simulink model "model"  (R2023a)
settings: Solver=VariableStepAuto  StartTime=0.0  StopTime=300  RelTol=1e-3
values from neighbouring files (symbols this model uses):
  r0 = unitToMJframe(r0)    [setup.m]
  r1 = unitToMJframe(r1)    [setup.m]
  r2 = unitToMJframe(r2)    [setup.m]
  r3 = unitToMJframe(r3)    [setup.m]
libraries: mjLib x4, sharedutil x4, sharedtransform x4
settings Model: PacingRate=4  Creator=manoj  LastModifiedBy=manoj

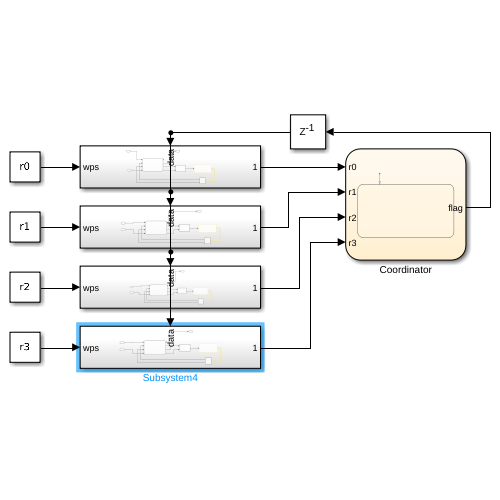
[thumbnail: Simulink's stored preview of the top-level diagram]
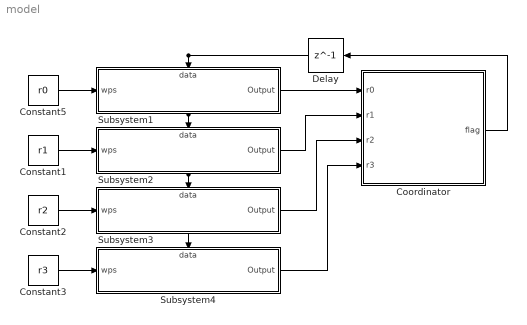
== system model ==
  Constant1 : Constant  Value=r1
  Constant2 : Constant  Value=r2
  Constant3 : Constant  Value=r3
  Constant5 : Constant  Value=r0
  Coordinator : Stateflow chart  TreatAsAtomicUnit=on
  Delay : Delay  DelayLength=1
  Subsystem1 : Subsystem
      settings: PortSchema="{\"entries\":[{\"content\":{\"sides\":[{\"content\":{\"connectorIds\":[\"In1\"]},\"type\":\"ConnectorPlacement.EquallySpacedRectSide\",\"uuid\":\"b8d0416c-6ae9-40e7-8587-4b4901c80a66\"},{\"content\":{\"connectorIds\":[\"Out1\"],\"side\":\"RIGHT\"},\"type\":\"ConnectorPlacement.EquallySpacedRectSide\",\"uuid\":\"eb8da2dc-17d6-409c-8414-2a6f0851cca1\"},{\"content\":{\"connectorIds\":[\"In2\"],\"side\":\"TOP\"},\"type\":\"ConnectorPlacement.EquallySpacedRectSide\",\"uuid\":\"007649e1-b7d1-46e6-9a26-22c717d3ea9f\"}]},\"type\":\"ConnectorPlacement.EquallySpacedConnector\",\"uuid\":\"2131bbaa-72b6-47e6-bef9-d625e80c0564\"}],\"packageUris\":[\"http://schema.mathworks.com/mf0/Connector/R2020b\"],\"version\":\"1.0\"}"
  Subsystem2 : Subsystem
      settings: PortSchema="{\"entries\":[{\"content\":{\"sides\":[{\"content\":{\"connectorIds\":[\"In1\"]},\"type\":\"ConnectorPlacement.EquallySpacedRectSide\",\"uuid\":\"b8d0416c-6ae9-40e7-8587-4b4901c80a66\"},{\"content\":{\"connectorIds\":[\"Out1\"],\"side\":\"RIGHT\"},\"type\":\"ConnectorPlacement.EquallySpacedRectSide\",\"uuid\":\"eb8da2dc-17d6-409c-8414-2a6f0851cca1\"},{\"content\":{\"connectorIds\":[\"In2\"],\"side\":\"TOP\"},\"type\":\"ConnectorPlacement.EquallySpacedRectSide\",\"uuid\":\"007649e1-b7d1-46e6-9a26-22c717d3ea9f\"}]},\"type\":\"ConnectorPlacement.EquallySpacedConnector\",\"uuid\":\"2131bbaa-72b6-47e6-bef9-d625e80c0564\"}],\"packageUris\":[\"http://schema.mathworks.com/mf0/Connector/R2020b\"],\"version\":\"1.0\"}"
  Subsystem3 : Subsystem
      settings: PortSchema="{\"entries\":[{\"content\":{\"sides\":[{\"content\":{\"connectorIds\":[\"In1\"]},\"type\":\"ConnectorPlacement.EquallySpacedRectSide\",\"uuid\":\"b8d0416c-6ae9-40e7-8587-4b4901c80a66\"},{\"content\":{\"connectorIds\":[\"Out1\"],\"side\":\"RIGHT\"},\"type\":\"ConnectorPlacement.EquallySpacedRectSide\",\"uuid\":\"eb8da2dc-17d6-409c-8414-2a6f0851cca1\"},{\"content\":{\"connectorIds\":[\"In2\"],\"side\":\"TOP\"},\"type\":\"ConnectorPlacement.EquallySpacedRectSide\",\"uuid\":\"007649e1-b7d1-46e6-9a26-22c717d3ea9f\"}]},\"type\":\"ConnectorPlacement.EquallySpacedConnector\",\"uuid\":\"2131bbaa-72b6-47e6-bef9-d625e80c0564\"}],\"packageUris\":[\"http://schema.mathworks.com/mf0/Connector/R2020b\"],\"version\":\"1.0\"}"
  Subsystem4 : Subsystem
      settings: PortSchema="{\"entries\":[{\"content\":{\"sides\":[{\"content\":{\"connectorIds\":[\"In1\"]},\"type\":\"ConnectorPlacement.EquallySpacedRectSide\",\"uuid\":\"b8d0416c-6ae9-40e7-8587-4b4901c80a66\"},{\"content\":{\"connectorIds\":[\"Out1\"],\"side\":\"RIGHT\"},\"type\":\"ConnectorPlacement.EquallySpacedRectSide\",\"uuid\":\"eb8da2dc-17d6-409c-8414-2a6f0851cca1\"},{\"content\":{\"connectorIds\":[\"In2\"],\"side\":\"TOP\"},\"type\":\"ConnectorPlacement.EquallySpacedRectSide\",\"uuid\":\"007649e1-b7d1-46e6-9a26-22c717d3ea9f\"}]},\"type\":\"ConnectorPlacement.EquallySpacedConnector\",\"uuid\":\"2131bbaa-72b6-47e6-bef9-d625e80c0564\"}],\"packageUris\":[\"http://schema.mathworks.com/mf0/Connector/R2020b\"],\"version\":\"1.0\"}"
  wires:
  Constant5/1 -> Subsystem1/1(wps)
  Constant1/1 -> Subsystem2/1(wps)
  Constant2/1 -> Subsystem3/1(wps)
  Constant3/1 -> Subsystem4/1(wps)
  Coordinator/1(flag) -> Delay/1
  Subsystem1/1(Output) -> Coordinator/1(r0)
  Subsystem2/1(Output) -> Coordinator/2(r1)
  Subsystem3/1(Output) -> Coordinator/3(r2)
  Subsystem4/1(Output) -> Coordinator/4(r3)
  Delay/1 -> Subsystem1/2(data), Subsystem4/2(data), Subsystem3/2(data), Subsystem2/2(data)

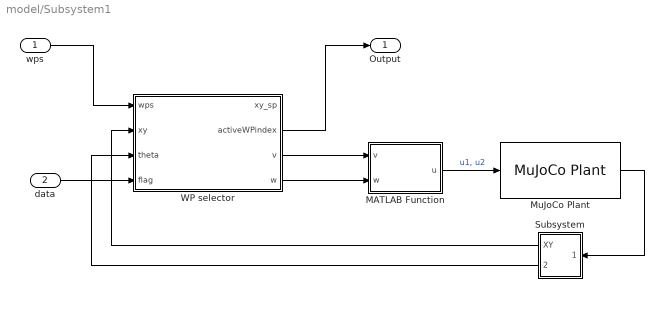
== system model/Subsystem1 ==
  wps : Inport
  data : Inport  Port=2
  MATLAB Function : MATLAB Function  TreatAsAtomicUnit=on
  MuJoCo Plant : mjLib/MuJoCo Plant  controlBus=[]  sensorBus=mj_bus_sensor_7979902499018342666  controlLength=[]  sensorLength=[]  rgbLength=[]  depthLength=[]  sampleTime=0.003  xmlFileRel=/home/manoj/work/courses/Multi_robot_centralized_planning/mujoco/mjxml/testClawbot.xml  xmlFile=/home/manoj/work/courses/Multi_robot_centralized_planning/mujoco/mjxml/testClawbot.xml  renderingType=Global  vsync=off  visualFPS=60  zoomLevel=1  znear=0.067117  zfar=335.5848  cameraSampleTime=0.020  rgbOutOption=on  depthOutOption=on  controlInterfaceType=Vector
      settings: SourceProductName=MuJoCo Simulator
  Subsystem : Subsystem
  WP selector : Stateflow chart  TreatAsAtomicUnit=on
      settings: PortSchema="{\"entries\":[{\"content\":{\"sides\":[{\"content\":{\"connectorIds\":[\"In1\",\"In2\",\"In3\",\"In4\"]},\"type\":\"ConnectorPlacement.EquallySpacedRectSide\",\"uuid\":\"c1ca6372-0066-48a0-9bc3-46210ce06805\"},{\"content\":{\"connectorIds\":[\"Out1\",\"Out2\",\"Out4\",\"Out3\"],\"side\":\"RIGHT\"},\"type\":\"ConnectorPlacement.EquallySpacedRectSide\",\"uuid\":\"5093fe73-baf8-4ce0-b37a-f548b4260345\"},{\"content\":{\"side\":\"TOP\"},\"type\":\"ConnectorPlacement.EquallySpacedRectSide\",\"uuid\":\"dd012d01-db43-40b1-a5e6-c3bf94706175\"}]},\"type\":\"ConnectorPlacement.EquallySpacedConnector\",\"uuid\":\"5c0fe838-8988-45a5-9c19-88c3336660b5\"}],\"packageUris\":[\"http://schema.mathworks.com/mf0/Connector/R2020b\"],\"version\":\"1.0\"}"
  Output : Outport
  wires:
  WP selector/4(v) -> MATLAB Function/1(v)
  MuJoCo Plant/1 -> Subsystem/1(In1)
  Subsystem/2(theta) -> WP selector/3(theta)
  WP selector/3(w) -> MATLAB Function/2(w)
  Subsystem/1(XY) -> WP selector/2(xy)
  MATLAB Function/1(u) -> MuJoCo Plant/1  "u1, u2"
  wps/1 -> WP selector/1(wps)
  WP selector/2(activeWPindex) -> Output/1
  data/1 -> WP selector/4(flag)

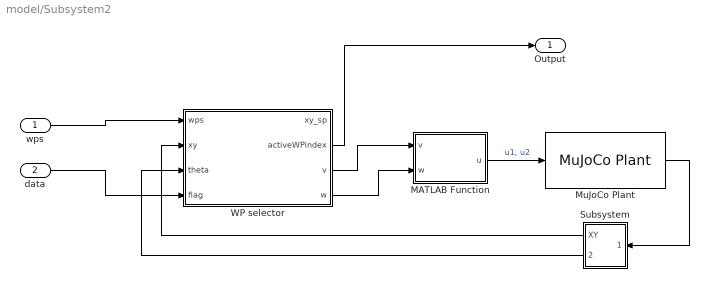
== system model/Subsystem2 ==
  wps : Inport
  data : Inport  Port=2
  MATLAB Function : MATLAB Function  TreatAsAtomicUnit=on
  MuJoCo Plant : mjLib/MuJoCo Plant  controlBus=[]  sensorBus=mj_bus_sensor_7979902499018342666  controlLength=[]  sensorLength=[]  rgbLength=[]  depthLength=[]  sampleTime=0.003  xmlFileRel=/home/manoj/work/courses/Multi_robot_centralized_planning/mujoco/mjxml/testClawbot1.xml  xmlFile=/home/manoj/work/courses/Multi_robot_centralized_planning/mujoco/mjxml/testClawbot1.xml  renderingType=Global  vsync=off  visualFPS=60  zoomLevel=1  znear=0.067117  zfar=335.5848  cameraSampleTime=0.020  rgbOutOption=on  depthOutOption=on  controlInterfaceType=Vector
      settings: SourceProductName=MuJoCo Simulator
  Subsystem : Subsystem
  WP selector : Stateflow chart  TreatAsAtomicUnit=on
      settings: PortSchema="{\"entries\":[{\"content\":{\"sides\":[{\"content\":{\"connectorIds\":[\"In1\",\"In2\",\"In3\",\"In4\"]},\"type\":\"ConnectorPlacement.EquallySpacedRectSide\",\"uuid\":\"c1ca6372-0066-48a0-9bc3-46210ce06805\"},{\"content\":{\"connectorIds\":[\"Out1\",\"Out2\",\"Out4\",\"Out3\"],\"side\":\"RIGHT\"},\"type\":\"ConnectorPlacement.EquallySpacedRectSide\",\"uuid\":\"5093fe73-baf8-4ce0-b37a-f548b4260345\"},{\"content\":{\"side\":\"TOP\"},\"type\":\"ConnectorPlacement.EquallySpacedRectSide\",\"uuid\":\"dd012d01-db43-40b1-a5e6-c3bf94706175\"}]},\"type\":\"ConnectorPlacement.EquallySpacedConnector\",\"uuid\":\"5c0fe838-8988-45a5-9c19-88c3336660b5\"}],\"packageUris\":[\"http://schema.mathworks.com/mf0/Connector/R2020b\"],\"version\":\"1.0\"}"
  Output : Outport
  wires:
  wps/1 -> WP selector/1(wps)
  MATLAB Function/1(u) -> MuJoCo Plant/1  "u1, u2"
  Subsystem/1(XY) -> WP selector/2(xy)
  WP selector/3(w) -> MATLAB Function/2(w)
  Subsystem/2(theta) -> WP selector/3(theta)
  MuJoCo Plant/1 -> Subsystem/1(In1)
  WP selector/4(v) -> MATLAB Function/1(v)
  WP selector/2(activeWPindex) -> Output/1
  data/1 -> WP selector/4(flag)

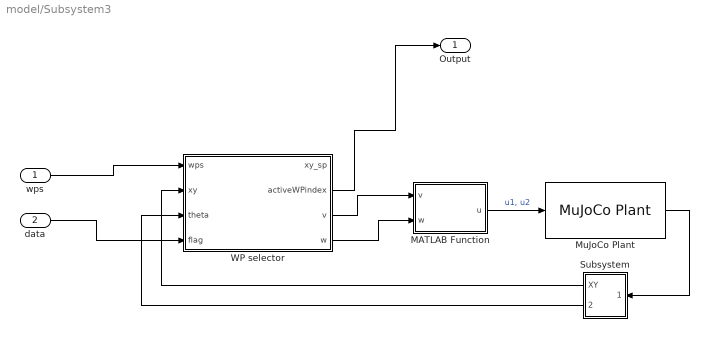
== system model/Subsystem3 ==
  wps : Inport
  data : Inport  Port=2
  MATLAB Function : MATLAB Function  TreatAsAtomicUnit=on
  MuJoCo Plant : mjLib/MuJoCo Plant  controlBus=[]  sensorBus=mj_bus_sensor_7979902499018342666  controlLength=[]  sensorLength=[]  rgbLength=[]  depthLength=[]  sampleTime=0.003  xmlFileRel=/home/manoj/work/courses/Multi_robot_centralized_planning/mujoco/mjxml/testClawbot2.xml  xmlFile=/home/manoj/work/courses/Multi_robot_centralized_planning/mujoco/mjxml/testClawbot2.xml  renderingType=Global  vsync=off  visualFPS=60  zoomLevel=1  znear=0.067117  zfar=335.5848  cameraSampleTime=0.020  rgbOutOption=on  depthOutOption=on  controlInterfaceType=Vector
      settings: SourceProductName=MuJoCo Simulator
  Subsystem : Subsystem
  WP selector : Stateflow chart  TreatAsAtomicUnit=on
      settings: PortSchema="{\"entries\":[{\"content\":{\"sides\":[{\"content\":{\"connectorIds\":[\"In1\",\"In2\",\"In3\",\"In4\"]},\"type\":\"ConnectorPlacement.EquallySpacedRectSide\",\"uuid\":\"c1ca6372-0066-48a0-9bc3-46210ce06805\"},{\"content\":{\"connectorIds\":[\"Out1\",\"Out2\",\"Out4\",\"Out3\"],\"side\":\"RIGHT\"},\"type\":\"ConnectorPlacement.EquallySpacedRectSide\",\"uuid\":\"5093fe73-baf8-4ce0-b37a-f548b4260345\"},{\"content\":{\"side\":\"TOP\"},\"type\":\"ConnectorPlacement.EquallySpacedRectSide\",\"uuid\":\"dd012d01-db43-40b1-a5e6-c3bf94706175\"}]},\"type\":\"ConnectorPlacement.EquallySpacedConnector\",\"uuid\":\"5c0fe838-8988-45a5-9c19-88c3336660b5\"}],\"packageUris\":[\"http://schema.mathworks.com/mf0/Connector/R2020b\"],\"version\":\"1.0\"}"
  Output : Outport
  wires:
  WP selector/4(v) -> MATLAB Function/1(v)
  MuJoCo Plant/1 -> Subsystem/1(In1)
  Subsystem/2(theta) -> WP selector/3(theta)
  WP selector/3(w) -> MATLAB Function/2(w)
  Subsystem/1(XY) -> WP selector/2(xy)
  MATLAB Function/1(u) -> MuJoCo Plant/1  "u1, u2"
  wps/1 -> WP selector/1(wps)
  WP selector/2(activeWPindex) -> Output/1
  data/1 -> WP selector/4(flag)

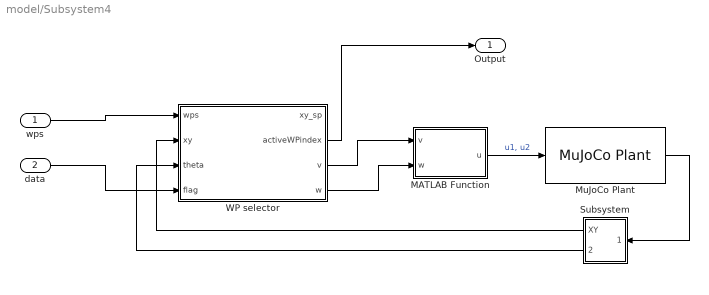
== system model/Subsystem4 ==
  wps : Inport
  data : Inport  Port=2
  MATLAB Function : MATLAB Function  TreatAsAtomicUnit=on
  MuJoCo Plant : mjLib/MuJoCo Plant  controlBus=[]  sensorBus=mj_bus_sensor_7979902499018342666  controlLength=[]  sensorLength=[]  rgbLength=[]  depthLength=[]  sampleTime=0.003  xmlFileRel=/home/manoj/work/courses/Multi_robot_centralized_planning/mujoco/mjxml/testClawbot3.xml  xmlFile=/home/manoj/work/courses/Multi_robot_centralized_planning/mujoco/mjxml/testClawbot3.xml  renderingType=Global  vsync=off  visualFPS=60  zoomLevel=1  znear=0.067117  zfar=335.5848  cameraSampleTime=0.020  rgbOutOption=on  depthOutOption=on  controlInterfaceType=Vector
      settings: SourceProductName=MuJoCo Simulator
  Subsystem : Subsystem
  WP selector : Stateflow chart  TreatAsAtomicUnit=on
      settings: PortSchema="{\"entries\":[{\"content\":{\"sides\":[{\"content\":{\"connectorIds\":[\"In1\",\"In2\",\"In3\",\"In4\"]},\"type\":\"ConnectorPlacement.EquallySpacedRectSide\",\"uuid\":\"c1ca6372-0066-48a0-9bc3-46210ce06805\"},{\"content\":{\"connectorIds\":[\"Out1\",\"Out2\",\"Out4\",\"Out3\"],\"side\":\"RIGHT\"},\"type\":\"ConnectorPlacement.EquallySpacedRectSide\",\"uuid\":\"5093fe73-baf8-4ce0-b37a-f548b4260345\"},{\"content\":{\"side\":\"TOP\"},\"type\":\"ConnectorPlacement.EquallySpacedRectSide\",\"uuid\":\"dd012d01-db43-40b1-a5e6-c3bf94706175\"}]},\"type\":\"ConnectorPlacement.EquallySpacedConnector\",\"uuid\":\"5c0fe838-8988-45a5-9c19-88c3336660b5\"}],\"packageUris\":[\"http://schema.mathworks.com/mf0/Connector/R2020b\"],\"version\":\"1.0\"}"
  Output : Outport
  wires:
  wps/1 -> WP selector/1(wps)
  MATLAB Function/1(u) -> MuJoCo Plant/1  "u1, u2"
  Subsystem/1(XY) -> WP selector/2(xy)
  WP selector/3(w) -> MATLAB Function/2(w)
  Subsystem/2(theta) -> WP selector/3(theta)
  MuJoCo Plant/1 -> Subsystem/1(In1)
  WP selector/4(v) -> MATLAB Function/1(v)
  WP selector/2(activeWPindex) -> Output/1
  data/1 -> WP selector/4(flag)

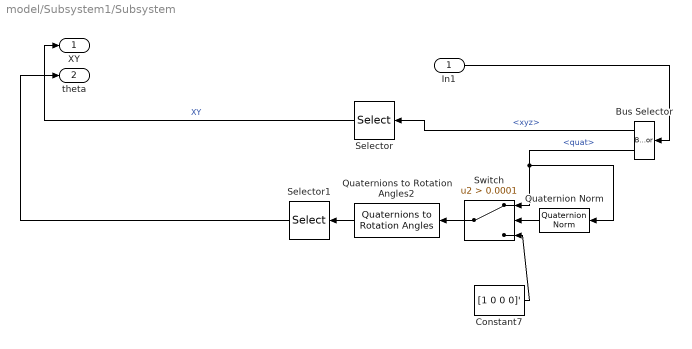
== system model/Subsystem1/Subsystem ==
  In1 : Inport
  Bus Selector : BusSelector  OutputSignals=xyz,quat
  Constant7 : Constant  Value=[1 0 0 0]'  VectorParams1D=off
  Quaternion Norm : sharedutil/Quaternion Norm  aMode=aMode
      settings: LibrarySourceBlock=|
      | aerolibutil/Quaternion
      | Norm
  Quaternions to Rotation Angles2 : sharedtransform/Quaternions to Rotation Angles  rotationOrder=ZYX  aMode=aMode
  Selector : Selector  InputPortWidth=3  IndexOptions=Index vector (dialog)  Indices=[1 2]  OutputSizes=1
  Selector1 : Selector  InputPortWidth=3  IndexOptions=Index vector (dialog)  Indices=1  OutputSizes=1
  Switch : Switch  Criteria=u2 > Threshold  Threshold=0.0001  SaturateOnIntegerOverflow=off  InputSameDT=off
  XY : Outport
  theta : Outport  Port=2
  wires:
  Quaternion Norm/1 -> Switch/2
  Selector1/1 -> theta/1
  Switch/1 -> Quaternions to Rotation Angles2/1
  Quaternions to Rotation Angles2/1 -> Selector1/1
  Bus Selector/2 -> Quaternion Norm/1, Switch/1  "<quat>"
  Bus Selector/1 -> Selector/1  "<xyz>"
  Constant7/1 -> Switch/3
  Selector/1 -> XY/1  "XY"
  In1/1 -> Bus Selector/1

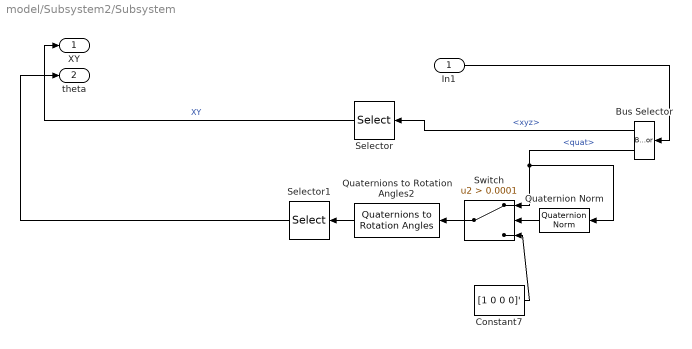
== system model/Subsystem2/Subsystem ==
  In1 : Inport
  Bus Selector : BusSelector  OutputSignals=xyz,quat
  Constant7 : Constant  Value=[1 0 0 0]'  VectorParams1D=off
  Quaternion Norm : sharedutil/Quaternion Norm  aMode=aMode
      settings: LibrarySourceBlock=|
      | aerolibutil/Quaternion
      | Norm
  Quaternions to Rotation Angles2 : sharedtransform/Quaternions to Rotation Angles  rotationOrder=ZYX  aMode=aMode
  Selector : Selector  InputPortWidth=3  IndexOptions=Index vector (dialog)  Indices=[1 2]  OutputSizes=1
  Selector1 : Selector  InputPortWidth=3  IndexOptions=Index vector (dialog)  Indices=1  OutputSizes=1
  Switch : Switch  Criteria=u2 > Threshold  Threshold=0.0001  SaturateOnIntegerOverflow=off  InputSameDT=off
  XY : Outport
  theta : Outport  Port=2
  wires:
  In1/1 -> Bus Selector/1
  Selector/1 -> XY/1  "XY"
  Constant7/1 -> Switch/3
  Bus Selector/1 -> Selector/1  "<xyz>"
  Bus Selector/2 -> Switch/1, Quaternion Norm/1  "<quat>"
  Quaternions to Rotation Angles2/1 -> Selector1/1
  Switch/1 -> Quaternions to Rotation Angles2/1
  Selector1/1 -> theta/1
  Quaternion Norm/1 -> Switch/2

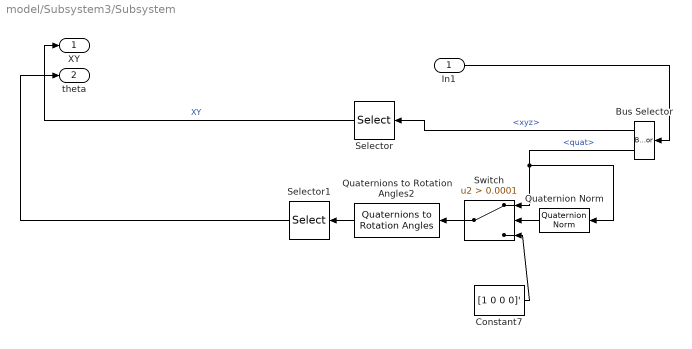
== system model/Subsystem3/Subsystem ==
  In1 : Inport
  Bus Selector : BusSelector  OutputSignals=xyz,quat
  Constant7 : Constant  Value=[1 0 0 0]'  VectorParams1D=off
  Quaternion Norm : sharedutil/Quaternion Norm  aMode=aMode
      settings: LibrarySourceBlock=|
      | aerolibutil/Quaternion
      | Norm
  Quaternions to Rotation Angles2 : sharedtransform/Quaternions to Rotation Angles  rotationOrder=ZYX  aMode=aMode
  Selector : Selector  InputPortWidth=3  IndexOptions=Index vector (dialog)  Indices=[1 2]  OutputSizes=1
  Selector1 : Selector  InputPortWidth=3  IndexOptions=Index vector (dialog)  Indices=1  OutputSizes=1
  Switch : Switch  Criteria=u2 > Threshold  Threshold=0.0001  SaturateOnIntegerOverflow=off  InputSameDT=off
  XY : Outport
  theta : Outport  Port=2
  wires:
  Quaternion Norm/1 -> Switch/2
  Selector1/1 -> theta/1
  Switch/1 -> Quaternions to Rotation Angles2/1
  Quaternions to Rotation Angles2/1 -> Selector1/1
  Bus Selector/2 -> Quaternion Norm/1, Switch/1  "<quat>"
  Bus Selector/1 -> Selector/1  "<xyz>"
  Constant7/1 -> Switch/3
  Selector/1 -> XY/1  "XY"
  In1/1 -> Bus Selector/1

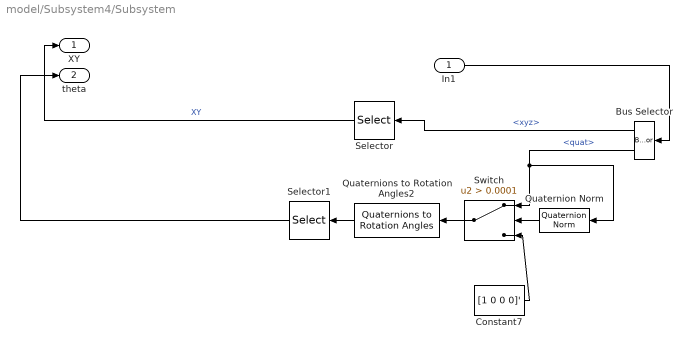
== system model/Subsystem4/Subsystem ==
  In1 : Inport
  Bus Selector : BusSelector  OutputSignals=xyz,quat
  Constant7 : Constant  Value=[1 0 0 0]'  VectorParams1D=off
  Quaternion Norm : sharedutil/Quaternion Norm  aMode=aMode
      settings: LibrarySourceBlock=|
      | aerolibutil/Quaternion
      | Norm
  Quaternions to Rotation Angles2 : sharedtransform/Quaternions to Rotation Angles  rotationOrder=ZYX  aMode=aMode
  Selector : Selector  InputPortWidth=3  IndexOptions=Index vector (dialog)  Indices=[1 2]  OutputSizes=1
  Selector1 : Selector  InputPortWidth=3  IndexOptions=Index vector (dialog)  Indices=1  OutputSizes=1
  Switch : Switch  Criteria=u2 > Threshold  Threshold=0.0001  SaturateOnIntegerOverflow=off  InputSameDT=off
  XY : Outport
  theta : Outport  Port=2
  wires:
  In1/1 -> Bus Selector/1
  Selector/1 -> XY/1  "XY"
  Constant7/1 -> Switch/3
  Bus Selector/1 -> Selector/1  "<xyz>"
  Bus Selector/2 -> Switch/1, Quaternion Norm/1  "<quat>"
  Quaternions to Rotation Angles2/1 -> Selector1/1
  Switch/1 -> Quaternions to Rotation Angles2/1
  Selector1/1 -> theta/1
  Quaternion Norm/1 -> Switch/2

== stateflow chart model/Subsystem3/WP selector ==
  state TRAVEL
    en, du:
    xy_err = xy_sp - xy';
    thetaExpected = atan2(xy_err(2), xy_err(1));
    thetaErr = thetaExpected - theta;
    if thetaErr>pi
    thetaErr = thetaErr -2*pi;
    end
    w = 6*thetaErr;
    if norm(xy_err)<0.1
    v = 0;
    else
    v = 3;
    end
  state TURN
    en, du:
    xy_err = xy_sp - xy';
    thetaExpected = atan2(xy_err(2), xy_err(1));
    thetaErr = thetaExpected - theta;
    if thetaErr>pi
    thetaErr = thetaErr -2*pi;
    end
    w = 6*thetaErr;
  state SWITCH
    en:
    activeWPindex = activeWPindex+1;
    %xy_sp =  [0 -0.5400]
  state WAIT_FOR_OTHERS
    en:
    xy_sp = wps(activeWPindex,:);
  state Terminate
  (default) -> SWITCH
  TURN -> TRAVEL : [norm(thetaErr)<3*pi/180]
  SWITCH -> WAIT_FOR_OTHERS [order 2]
  WAIT_FOR_OTHERS -> TURN : [flag==true]
  TRAVEL -> SWITCH : [norm(xy_err)<0.1]
  SWITCH -> Terminate [order 1] : [activeWPindex>7]
  data: wps input; xy_sp output; activeWPindex output =1; thetaExpected local; thetaErr local; w output; v output; xy input; theta input; xy_err local; flag input

== matlab function model/Subsystem4/MATLAB Function ==
  data: v input; u output; w input
function u = fcn(v, w)

u = [v+w, v-w]';

== stateflow chart model/Subsystem4/WP selector ==
  state TRAVEL
    en, du:
    xy_err = xy_sp - xy';
    thetaExpected = atan2(xy_err(2), xy_err(1));
    thetaErr = thetaExpected - theta;
    if thetaErr>pi
    thetaErr = thetaErr -2*pi;
    end
    w = 6*thetaErr;
    if norm(xy_err)<0.1
    v = 0;
    else
    v = -3;
    end
  state TURN
    en, du:
    xy_err = xy_sp - xy';
    thetaExpected = atan2(xy_err(2), xy_err(1));
    thetaErr = thetaExpected - theta;
    if thetaErr>pi
    thetaErr = thetaErr -2*pi;
    end
    w = 6*thetaErr;
  state SWITCH
    en:
    activeWPindex = activeWPindex+1;
    %xy_sp =  [0 -0.5400]
  state WAIT_FOR_OTHERS
    en:
    xy_sp = wps(activeWPindex,:);
  state Terminate
  (default) -> SWITCH
  TURN -> TRAVEL : [norm(thetaErr)<3*pi/180]
  WAIT_FOR_OTHERS -> TURN : [flag==true]
  SWITCH -> WAIT_FOR_OTHERS [order 2]
  TRAVEL -> SWITCH : [norm(xy_err)<0.1]
  SWITCH -> Terminate [order 1] : [activeWPindex>7]
  data: wps input; xy_sp output; activeWPindex output =1; thetaExpected local; thetaErr local; w output; v output; xy input; theta input; xy_err local; flag input

== stateflow chart model/Coordinator ==
  state COUNTER
    en, du:
    if var([r0, r1, r2, r3]) < 0.01
    flag = true;
    else
    flag = false;
    end
  (default) -> COUNTER
  data: flag output; r0 input; r1 input; r2 input; r3 input

== matlab function model/Subsystem2/MATLAB Function ==
  data: v input; u output; w input
function u = fcn(v, w)

u = [v+w, v-w]';

== matlab function model/Subsystem1/MATLAB Function ==
  data: v input; u output; w input
function u = fcn(v, w)

u = [v+w, v-w]';

== stateflow chart model/Subsystem1/WP selector ==
  state TURN
    en, du:
    xy_err = xy_sp - xy';
    thetaExpected = atan2(xy_err(2), xy_err(1));
    thetaErr = thetaExpected - theta;
    if thetaErr>pi
    thetaErr = thetaErr -2*pi;
    end
    w = 6*thetaErr;
  state TRAVEL
    en, du:
    xy_err = xy_sp - xy';
    thetaExpected = atan2(xy_err(2), xy_err(1));
    thetaErr = thetaExpected - theta;
    if thetaErr>pi
    thetaErr = thetaErr -2*pi;
    end
    w = 6*thetaErr;
    if norm(xy_err)<0.1
    v = 0;
    else
    v = -3;
    end
  state SWITCH
    en:
    activeWPindex = activeWPindex+1;
    %xy_sp =  [0 -0.5400]
  state WAIT_FOR_OTHERS
    en:
    xy_sp = wps(activeWPindex,:);
  state Terminate
  (default) -> SWITCH
  TURN -> TRAVEL : [norm(thetaErr)<3*pi/180]
  SWITCH -> WAIT_FOR_OTHERS [order 2]
  WAIT_FOR_OTHERS -> TURN : [flag==true]
  TRAVEL -> SWITCH : [norm(xy_err)<0.1]
  SWITCH -> Terminate [order 1] : [activeWPindex>7]
  data: wps input; xy_sp output; activeWPindex output =1; thetaExpected local; thetaErr local; w output; v output; xy input; theta input; xy_err local; flag input

== stateflow chart model/Subsystem2/WP selector ==
  state TURN
    en, du:
    xy_err = xy_sp - xy';
    thetaExpected = atan2(xy_err(2), xy_err(1));
    thetaErr = thetaExpected - theta;
    if thetaErr>pi
    thetaErr = thetaErr -2*pi;
    end
    w = 6*thetaErr;
  state TRAVEL
    en, du:
    xy_err = xy_sp - xy';
    thetaExpected = atan2(xy_err(2), xy_err(1));
    thetaErr = thetaExpected - theta;
    if thetaErr>pi
    thetaErr = thetaErr -2*pi;
    end
    w = 6*thetaErr;
    if norm(xy_err)<0.1
    v = 0;
    else
    v = -3;
    end
  state SWITCH
    en:
    activeWPindex = activeWPindex+1;
    %xy_sp =  [0 -0.5400]
  state WAIT_FOR_OTHERS
    en:
    xy_sp = wps(activeWPindex,:);
  state Terminate
  (default) -> SWITCH
  TURN -> TRAVEL : [norm(thetaErr)<3*pi/180]
  SWITCH -> WAIT_FOR_OTHERS [order 2]
  WAIT_FOR_OTHERS -> TURN : [flag==true]
  TRAVEL -> SWITCH : [norm(xy_err)<0.1]
  SWITCH -> Terminate [order 1] : [activeWPindex>7]
  data: wps input; xy_sp output; activeWPindex output =1; thetaExpected local; thetaErr local; w output; v output; xy input; theta input; xy_err local; flag input

== matlab function model/Subsystem3/MATLAB Function ==
  data: v input; u output; w input
function u = fcn(v, w)

u = [v+w, v-w]';
